simulink model "Callum_Model"  (R2018a)
settings: Solver=VariableStepAuto  StartTime=0.0  StopTime=10.0  RelTol=1e-3
model workspace (MAT data in the model file):
  x = Simulink.Parameter
  x.DataType = 'auto'
  x.Dimensions = [0 0]
settings Model: Creator=wjf14  LastModifiedBy=wjf14

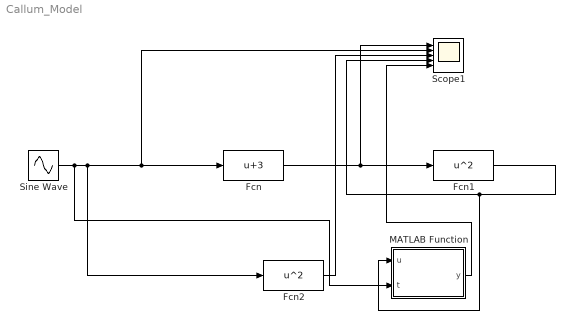
== system Callum_Model ==
  Fcn : Fcn  Expr=u+3
  Fcn1 : Fcn  Expr=u^2
  Fcn2 : Fcn  Expr=u^2
  MATLAB Function : MATLAB Function  TreatAsAtomicUnit=on
  Scope1 : Scope  NumInputPorts=5
  Sine Wave : Sin  SampleTime=0
  wires:
  Sine Wave/1 -> MATLAB Function/2(t), Fcn2/1, Scope1/2, Fcn/1
  Fcn/1 -> Fcn1/1, Scope1/1
  Fcn1/1 -> MATLAB Function/1(u), Scope1/4
  Fcn2/1 -> Scope1/3
  MATLAB Function/1(y) -> Scope1/5

== matlab function Callum_Model/MATLAB Function ==
  data: u input; y output; t input
function y  = fcn(u, t)

y = u+t;
end
